simulink model "RUL_system_DL"  (R2022b)
settings: Solver=VariableStepAuto  StartTime=0.0  StopTime=XTest_signal.Time(end)  RelTol=1e-3
settings Model: Creator=tshintai  LastModifiedBy=tshintai
settings DebuggingCC: UnconnectedInputMsg=warning  UnconnectedOutputMsg=warning  UnconnectedLineMsg=warning
settings ModelReferenceCC: EnableRefExpFcnMdlSchedulingChecks=on  PropagateVarSize=During execution
settings RTWCC: DLArmComputeVersion=19.05

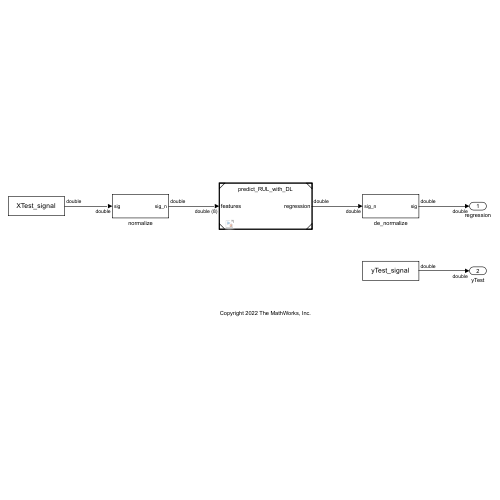
[thumbnail: Simulink's stored preview of the top-level diagram]
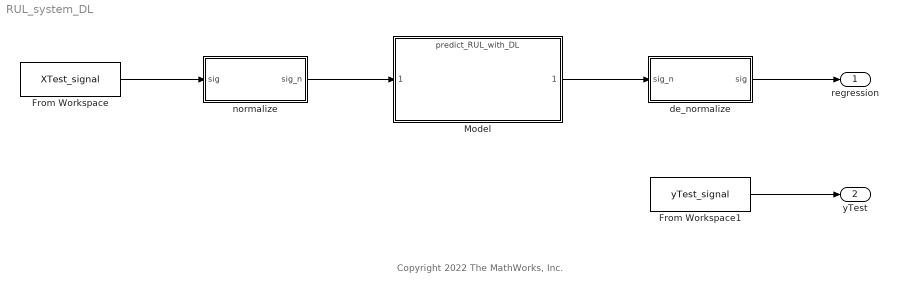
== system RUL_system_DL ==
  note: Copyright 2022 The MathWorks, Inc.
  From Workspace : FromWorkspace  VariableName=XTest_signal  SampleTime=1  Interpolate=off  OutputAfterFinalValue=Holding final value
  From Workspace1 : FromWorkspace  VariableName=yTest_signal  SampleTime=1  Interpolate=off  OutputAfterFinalValue=Holding final value
  Model : ModelReference  ModelNameDialog=predict_RUL_with_DL  SimulationMode=Normal  ModelReferenceVersion=3.1
  de_normalize : Subsystem
  normalize : Subsystem
  regression : Outport
  yTest : Outport  Port=2
  wires:
  From Workspace/1 -> normalize/1(sig)
  Model/1 -> de_normalize/1(sig_n)
  From Workspace1/1 -> yTest/1
  normalize/1(sig_n) -> Model/1
  de_normalize/1(sig) -> regression/1

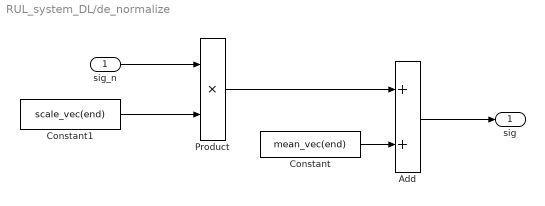
== system RUL_system_DL/de_normalize ==
  sig_n : Inport
  Add : Sum
  Constant : Constant  Value=mean_vec(end)
  Constant1 : Constant  Value=scale_vec(end)
  Product : Product
  sig : Outport
  wires:
  Add/1 -> sig/1
  Constant/1 -> Add/2
  sig_n/1 -> Product/1
  Constant1/1 -> Product/2
  Product/1 -> Add/1

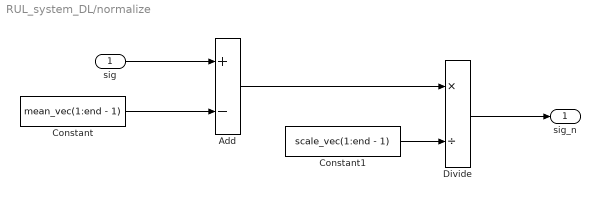
== system RUL_system_DL/normalize ==
  sig : Inport
  Add : Sum  Inputs=+-
  Constant : Constant  Value=mean_vec(1:end - 1)
  Constant1 : Constant  Value=scale_vec(1:end - 1)
  Divide : Product  Inputs=*/
  sig_n : Outport
  wires:
  sig/1 -> Add/1
  Constant/1 -> Add/2
  Add/1 -> Divide/1
  Constant1/1 -> Divide/2
  Divide/1 -> sig_n/1
